simulink model "sampleModel1804_5_sub_sub"  (R2023a)
settings: Solver=VariableStepAuto  StartTime=0.0  StopTime=10.0  RelTol=1e-3
libraries: hdlsllib x5, simulink x1
settings Model: Creator=user1  LastModifiedBy=user1

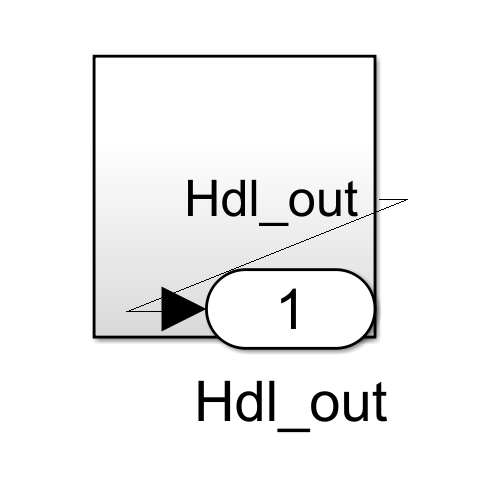
[thumbnail: Simulink's stored preview of the top-level diagram]
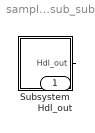
== system sampleModel1804_5_sub_sub ==
  Subsystem : Subsystem
  Hdl_out : Outport  OutDataTypeStr=uint8
  wires:
  Subsystem/1(Hdl_out) -> Hdl_out/1

== system sampleModel1804_5_sub_sub/Subsystem ==
  Subsystem : Subsystem
  Hdl_out : Outport  OutDataTypeStr=uint8

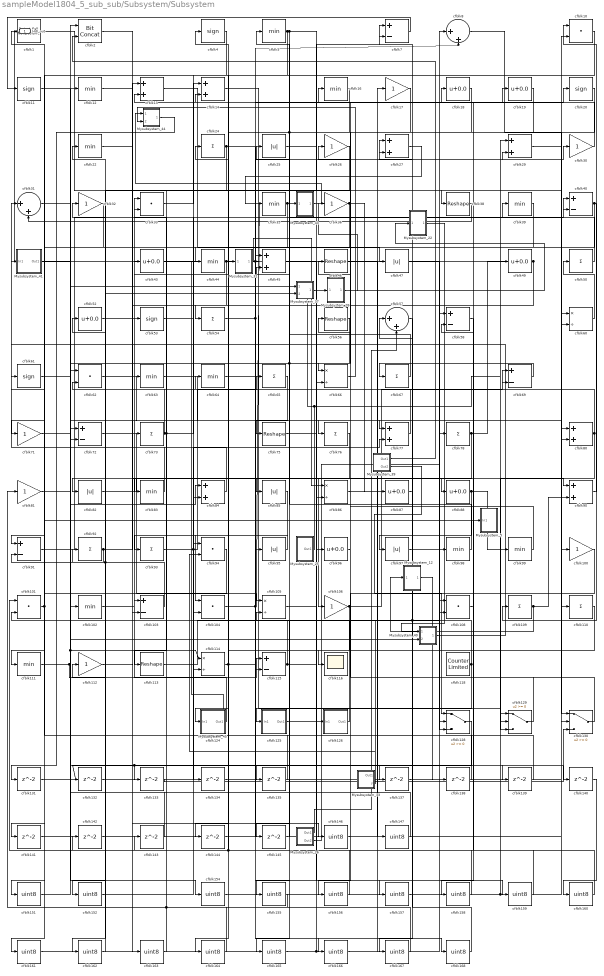
== system sampleModel1804_5_sub_sub/Subsystem/Subsystem ==
  Mysubsystem_12 : Subsystem  TreatAsAtomicUnit=on  RTWFcnName=Mysubsystem_12
      settings: RTWFcnNameOpts=User specified  RTWFileNameOpts=Use function name
  Mysubsystem_22 : Subsystem  TreatAsAtomicUnit=on  RTWFcnName=Mysubsystem_22
      settings: RTWFcnNameOpts=User specified  RTWFileNameOpts=Use function name
  Mysubsystem_25 : Subsystem  TreatAsAtomicUnit=on  RTWFcnName=Mysubsystem_25
      settings: RTWFcnNameOpts=User specified  RTWFileNameOpts=Use function name
  Mysubsystem_26 : Subsystem  TreatAsAtomicUnit=on  RTWFcnName=Mysubsystem_26
      settings: RTWFcnNameOpts=User specified  RTWFileNameOpts=Use function name
  Mysubsystem_28 : Subsystem  TreatAsAtomicUnit=on  RTWFcnName=Mysubsystem_28
      settings: RTWFcnNameOpts=User specified  RTWFileNameOpts=Use function name
  Mysubsystem_31 : Subsystem  TreatAsAtomicUnit=on  RTWFcnName=Mysubsystem_31
      settings: RTWFcnNameOpts=User specified  RTWFileNameOpts=Use function name
  Mysubsystem_33 : Subsystem  TreatAsAtomicUnit=on  RTWFcnName=Mysubsystem_33
      settings: RTWFcnNameOpts=User specified  RTWFileNameOpts=Use function name
  Mysubsystem_37 : Subsystem  TreatAsAtomicUnit=on  RTWFcnName=Mysubsystem_37
      settings: RTWFcnNameOpts=User specified  RTWFileNameOpts=Use function name
  Mysubsystem_39 : Subsystem  TreatAsAtomicUnit=on  RTWFcnName=Mysubsystem_39
      settings: RTWFcnNameOpts=User specified  RTWFileNameOpts=Use function name
  Mysubsystem_40 : Subsystem  TreatAsAtomicUnit=on  RTWFcnName=Mysubsystem_40
      settings: RTWFcnNameOpts=User specified  RTWFileNameOpts=Use function name
  Mysubsystem_41 : Subsystem  TreatAsAtomicUnit=on  RTWFcnName=Mysubsystem_41
      settings: RTWFcnNameOpts=User specified  RTWFileNameOpts=Use function name
  Mysubsystem_43 : Subsystem  TreatAsAtomicUnit=on  RTWFcnName=Mysubsystem_43
      settings: RTWFcnNameOpts=User specified  RTWFileNameOpts=Use function name
  Mysubsystem_44 : Subsystem  TreatAsAtomicUnit=on  RTWFcnName=Mysubsystem_44
      settings: RTWFcnNameOpts=User specified  RTWFileNameOpts=Use function name
  Mysubsystem_45 : Subsystem  TreatAsAtomicUnit=on  RTWFcnName=Mysubsystem_45
      settings: RTWFcnNameOpts=User specified  RTWFileNameOpts=Use function name
  Mysubsystem_5 : Subsystem  TreatAsAtomicUnit=on  RTWFcnName=Mysubsystem_5
      settings: RTWFcnNameOpts=User specified  RTWFileNameOpts=Use function name
  cfblk1 : hdlsllib/Logic and Bit Operations/Detect Fall Nonpositive  vinit=0  OutDataTypeStr=uint8
  cfblk{10,33,62,94,101,104,108} (7 alike) : DotProduct  OutDataTypeStr=uint8
  cfblk{17,26,30,32,36,71,81,100,106,112} (10 alike) : Gain  OutDataTypeStr=uint8
  cfblk{5,12,16,22,35,39,44,63..64,83,98..99,102,111} (14 alike) : MinMax  OutDataTypeStr=uint8
  cfblk{7,40,58,69,72,91,103,115} (8 alike) : Sum  Inputs=+-  OutDataTypeStr=uint8
  cfblk{60,66,86,105,114} (5 alike) : Product  Inputs=*/  OutDataTypeStr=uint8  RndMeth=Zero  SaturateOnIntegerOverflow=on
  cfblk{24,50,54,65,67,73,76,78,92..93,109..110} (12 alike) : Sum  Inputs=+  OutDataTypeStr=uint8
  cfblk{4,11,20,53,61} (5 alike) : Signum
  cfblk{38,46,56,75,113} (5 alike) : Reshape
  cfblk116 : Scope
  cfblk118 : hdlsllib/Sources/Counter Limited  uplimit=7  tsamp=-1
  cfblk124 : Subsystem
      settings: LibrarySourceBlock=|
      | hdlsllib/Ports &
      | Subsystems/Subsystem
  cfblk125 : Subsystem
      settings: LibrarySourceBlock=|
      | hdlsllib/Ports &
      | Subsystems/Subsystem
  cfblk126 : Subsystem
      settings: LibrarySourceBlock=|
      | hdlsllib/Ports &
      | Subsystems/Subsystem
  cfblk128 : Switch  OutDataTypeStr=uint8  SaturateOnIntegerOverflow=off  InputSameDT=off
  cfblk129 : Switch  OutDataTypeStr=uint8  SaturateOnIntegerOverflow=off  InputSameDT=off
  cfblk{13..14,27,29,45,77,80,84,90} (9 alike) : Sum  OutDataTypeStr=uint8
  cfblk130 : Switch  OutDataTypeStr=uint8  SaturateOnIntegerOverflow=off  InputSameDT=off
  cfblk{131..135,137..145} (14 alike) : Delay  SampleTime=1
  cfblk{146..147,151..152,154..168} (19 alike) : DataTypeConversion  OutDataTypeStr=uint8  SaturateOnIntegerOverflow=off  RndMeth=Floor
  cfblk{18..19,43,49,52,87..88,96} (8 alike) : Bias  Bias=0.0  SaturateOnIntegerOverflow=off
  cfblk2 : hdlsllib/Logic and Bit Operations/Bit Concat  numInputs=2
  cfblk{25,47,82,85,95,97} (6 alike) : Abs  OutDataTypeStr=uint8  SaturateOnIntegerOverflow=off
  cfblk31 : Sum  Inputs=|++  OutDataTypeStr=uint8
  cfblk57 : Sum  Inputs=|++  OutDataTypeStr=uint8
  cfblk8 : Sum  Inputs=|++  OutDataTypeStr=uint8
  Hdl_out : Outport  OutDataTypeStr=uint8
  wires:
  Mysubsystem_45/1(Out1) -> Mysubsystem_31/1(In1)
  Mysubsystem_44/1(Out1) -> cfblk131/1
  cfblk66/1 -> Mysubsystem_44/2(In2)
  Mysubsystem_43/1(Out1) -> Mysubsystem_44/1(In1)
  cfblk27/1 -> Mysubsystem_43/1(In1)
  Mysubsystem_41/1(Out1) -> Mysubsystem_40/2(In2)
  Mysubsystem_40/1(Out1) -> Mysubsystem_41/1(In1)
  Mysubsystem_22/1(Out1) -> Mysubsystem_40/1(In1)
  Mysubsystem_39/2(Out2) -> cfblk128/1
  Mysubsystem_39/1(Out1) -> cfblk2/2
  Mysubsystem_37/1(Out1) -> Mysubsystem_22/1(In1)
  cfblk31/1 -> Mysubsystem_37/1(In1)
  Mysubsystem_33/2(y) -> cfblk101/2
  Mysubsystem_33/1(Out1) -> cfblk94/2
  Mysubsystem_31/1(Out1) -> cfblk86/1
  Mysubsystem_28/1(Out1) -> cfblk36/1
  Mysubsystem_26/2(Out2) -> cfblk78/1
  Mysubsystem_26/1(Out1) -> cfblk57/2
  Mysubsystem_25/1(Out1) -> cfblk40/2, Mysubsystem_28/1(In1)
  Mysubsystem_12/1(Out1) -> cfblk138/1
  cfblk168/1 -> cfblk57/1
  cfblk64/1 -> cfblk168/1
  cfblk167/1 -> cfblk143/1, cfblk142/1
  cfblk166/1 -> cfblk17/1
  cfblk165/1 -> cfblk126/1(In1)
  cfblk17/1 -> cfblk165/1
  cfblk164/1 -> cfblk112/1
  cfblk163/1 -> cfblk33/2
  cfblk112/1 -> cfblk163/1
  cfblk162/1 -> cfblk32/1
  cfblk26/1 -> cfblk162/1
  cfblk161/1 -> cfblk108/2, cfblk96/1
  cfblk160/1 -> cfblk58/2
  cfblk140/1 -> cfblk160/1
  cfblk159/1 -> cfblk58/1
  cfblk158/1 -> cfblk62/2
  cfblk58/1 -> cfblk158/1
  cfblk157/1 -> cfblk100/1
  cfblk156/1 -> cfblk64/1, cfblk101/1
  cfblk155/1 -> cfblk81/1
  cfblk154/1 -> cfblk10/2, cfblk29/1
  cfblk152/1 -> cfblk94/1
  cfblk39/1 -> cfblk152/1
  cfblk151/1 -> cfblk102/1
  cfblk94/1 -> cfblk151/1
  cfblk147/1 -> cfblk2/1
  cfblk46/1 -> cfblk147/1
  cfblk146/1 -> cfblk108/1
  cfblk2/1 -> cfblk146/1
  cfblk145/1 -> cfblk105/2
  cfblk144/1 -> cfblk80/1
  cfblk110/1 -> cfblk144/1
  cfblk143/1 -> cfblk72/1
  cfblk142/1 -> cfblk45/1
  cfblk141/1 -> cfblk114/2
  cfblk139/1 -> cfblk1/1
  cfblk138/1 -> cfblk14/2
  cfblk137/1 -> cfblk129/1
  cfblk22/1 -> cfblk137/1
  cfblk135/1 -> cfblk62/1
  cfblk134/1 -> cfblk60/1
  cfblk43/1 -> cfblk134/1
  cfblk133/1 -> cfblk130/3
  cfblk132/1 -> cfblk115/2
  cfblk131/1 -> cfblk130/2
  cfblk63/1 -> cfblk95/1
  cfblk73/1 -> cfblk40/1, cfblk113/1, cfblk63/1
  cfblk45/1 -> cfblk129/2
  cfblk65/1 -> cfblk75/1
  cfblk100/1 -> cfblk156/1
  cfblk114/1 -> cfblk24/1, cfblk157/1
  cfblk101/1 -> Mysubsystem_5/1(In1), cfblk141/1
  cfblk97/1 -> cfblk98/1
  cfblk87/1 -> cfblk27/2
  cfblk24/1 -> cfblk83/1, cfblk140/1
  cfblk113/1 -> cfblk8/1
  cfblk95/1 -> cfblk93/1
  cfblk25/1 -> cfblk29/2
  cfblk50/1 -> cfblk25/1
  cfblk80/1 -> cfblk4/1, cfblk129/3
  cfblk98/1 -> cfblk45/2
  cfblk109/1 -> Mysubsystem_12/1(In1), cfblk90/2
  cfblk105/1 -> cfblk20/1
  cfblk38/1 -> cfblk31/2
  cfblk32/1 -> cfblk161/1
  cfblk57/1 -> cfblk167/1
  cfblk53/1 -> cfblk88/1
  cfblk11/1 -> cfblk77/1
  cfblk52/1 -> cfblk86/2
  cfblk128/1 -> cfblk132/1, cfblk133/1
  cfblk125/1(Out1) -> cfblk66/2
  cfblk29/1 -> cfblk130/1
  cfblk67/1 -> cfblk5/1
  cfblk71/1 -> cfblk12/1
  cfblk82/1 -> cfblk90/1
  cfblk77/1 -> cfblk22/1
  cfblk19/1 -> cfblk54/1
  cfblk8/1 -> cfblk110/1
  cfblk1/1 -> cfblk60/2
  cfblk88/1 -> cfblk97/1, cfblk99/1
  cfblk99/1 -> cfblk46/1
  cfblk12/1 -> cfblk53/1
  cfblk106/1 -> cfblk69/2, cfblk116/1
  cfblk84/1 -> cfblk73/1
  cfblk90/1 -> cfblk10/1
  cfblk124/1(Out1) -> cfblk103/1
  cfblk10/1 -> cfblk124/1(In1)
  cfblk60/1 -> cfblk50/1
  cfblk93/1 -> cfblk65/1, cfblk77/2
  cfblk96/1 -> cfblk56/1
  cfblk40/1 -> cfblk109/1, cfblk91/1
  cfblk86/1 -> cfblk69/1
  cfblk103/1 -> Mysubsystem_37/2(In2), cfblk61/1
  cfblk47/1 -> cfblk128/3
  cfblk115/1 -> cfblk92/1, cfblk159/1
  cfblk72/1 -> cfblk105/1
  cfblk33/1 -> cfblk14/1
  cfblk49/1 -> cfblk104/2, Hdl_out/1
  cfblk16/1 -> cfblk85/1
  cfblk111/1 -> cfblk115/1, cfblk84/1
  cfblk18/1 -> cfblk66/1
  cfblk76/1 -> cfblk106/1
  cfblk44/1 -> cfblk128/2, cfblk8/2, cfblk103/2
  cfblk78/1 -> cfblk82/1, cfblk49/1
  cfblk69/1 -> cfblk67/1
  cfblk30/1 -> cfblk13/2
  cfblk4/1 -> cfblk71/1
  cfblk56/1 -> cfblk72/2, cfblk135/1
  cfblk129/1 -> cfblk26/1
  cfblk85/1 -> cfblk104/1
  cfblk81/1 -> cfblk154/1
  cfblk5/1 -> cfblk38/1, cfblk125/1(In1), cfblk84/2
  cfblk7/1 -> cfblk11/1
  cfblk75/1 -> cfblk7/1
  cfblk36/1 -> cfblk44/1, cfblk87/1
  cfblk61/1 -> cfblk114/1, cfblk139/1
  cfblk108/1 -> cfblk18/1
  cfblk54/1 -> cfblk30/1, cfblk166/1
  cfblk83/1 -> cfblk31/1
  cfblk20/1 -> cfblk145/1, cfblk164/1
  cfblk62/1 -> cfblk80/2
  cfblk118/1 -> cfblk52/1, cfblk7/2, cfblk155/1
  cfblk35/1 -> cfblk27/1, cfblk111/1
  cfblk92/1 -> cfblk13/1, cfblk91/2
  cfblk91/1 -> cfblk39/1
  cfblk130/1 -> cfblk16/1
  cfblk104/1 -> cfblk35/1, cfblk19/1
  cfblk102/1 -> cfblk43/1
  cfblk126/1(Out1) -> cfblk33/1
  cfblk14/1 -> cfblk76/1
  cfblk13/1 -> cfblk47/1

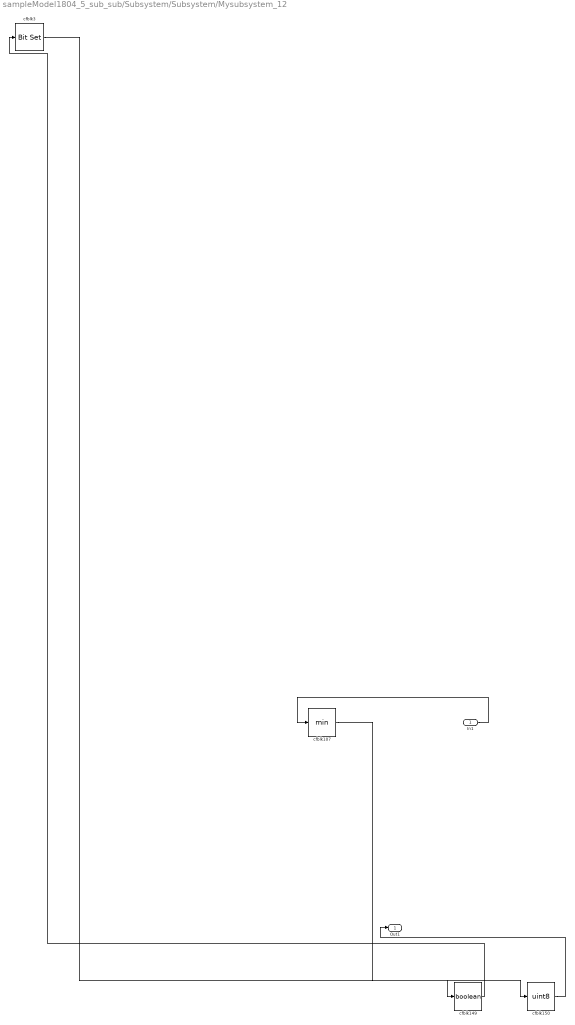
== system sampleModel1804_5_sub_sub/Subsystem/Subsystem/Mysubsystem_12 ==
  In1 : Inport
  cfblk107 : MinMax
  cfblk149 : DataTypeConversion  OutDataTypeStr=boolean  SaturateOnIntegerOverflow=off  RndMeth=Floor
  cfblk150 : DataTypeConversion  OutDataTypeStr=uint8  SaturateOnIntegerOverflow=off  RndMeth=Floor
  cfblk3 : simulink/Logic and Bit Operations/Bit Set  iBit=0
      settings: LibrarySourceBlock=|
      | hdlsllib/Logic and Bit
      | Operations/Bit Set
  Out1 : Outport
  wires:
  cfblk150/1 -> Out1/1
  cfblk3/1 -> cfblk150/1
  cfblk149/1 -> cfblk3/1
  cfblk107/1 -> cfblk149/1
  In1/1 -> cfblk107/1

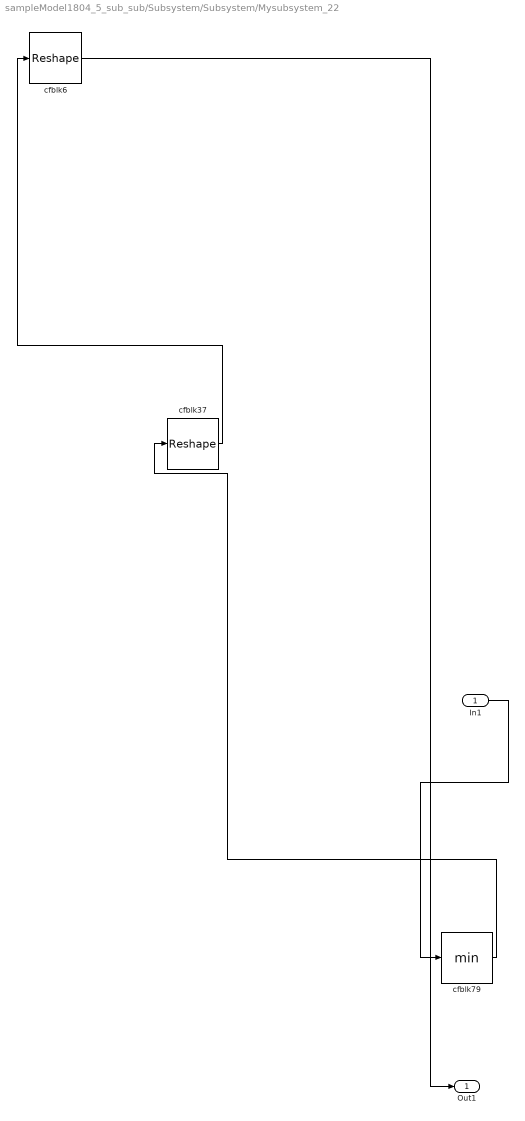
== system sampleModel1804_5_sub_sub/Subsystem/Subsystem/Mysubsystem_22 ==
  In1 : Inport
  cfblk37 : Reshape
  cfblk6 : Reshape
  cfblk79 : MinMax
  Out1 : Outport
  wires:
  cfblk37/1 -> cfblk6/1
  cfblk79/1 -> cfblk37/1
  In1/1 -> cfblk79/1
  cfblk6/1 -> Out1/1

== system sampleModel1804_5_sub_sub/Subsystem/Subsystem/Mysubsystem_25 ==
  cfblk123 : Constant  SampleTime=-1
  cfblk68 : Reshape
  Out1 : Outport
  wires:
  cfblk123/1 -> cfblk68/1
  cfblk68/1 -> Out1/1

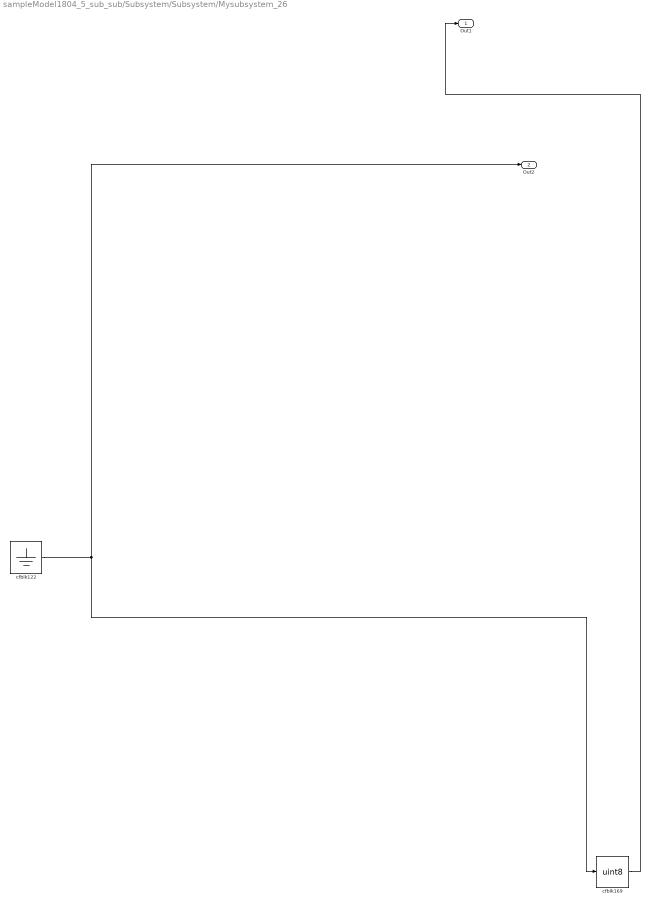
== system sampleModel1804_5_sub_sub/Subsystem/Subsystem/Mysubsystem_26 ==
  cfblk122 : Ground
  cfblk169 : DataTypeConversion  OutDataTypeStr=uint8  SaturateOnIntegerOverflow=off  RndMeth=Floor
  Out1 : Outport
  Out2 : Outport  Port=2
  wires:
  cfblk122/1 -> Out2/1, cfblk169/1
  cfblk169/1 -> Out1/1

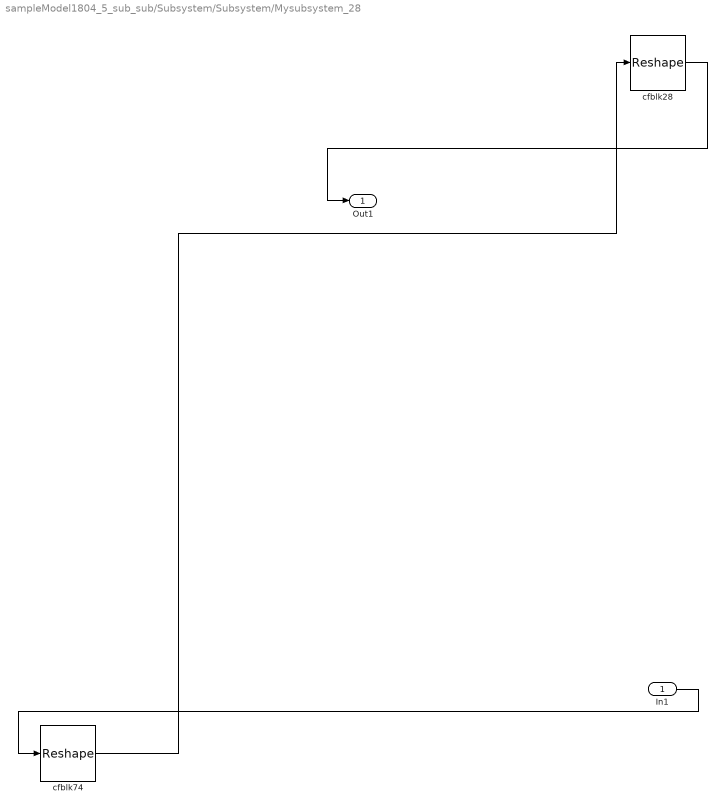
== system sampleModel1804_5_sub_sub/Subsystem/Subsystem/Mysubsystem_28 ==
  In1 : Inport
  cfblk28 : Reshape
  cfblk74 : Reshape
  Out1 : Outport
  wires:
  cfblk74/1 -> cfblk28/1
  cfblk28/1 -> Out1/1
  In1/1 -> cfblk74/1

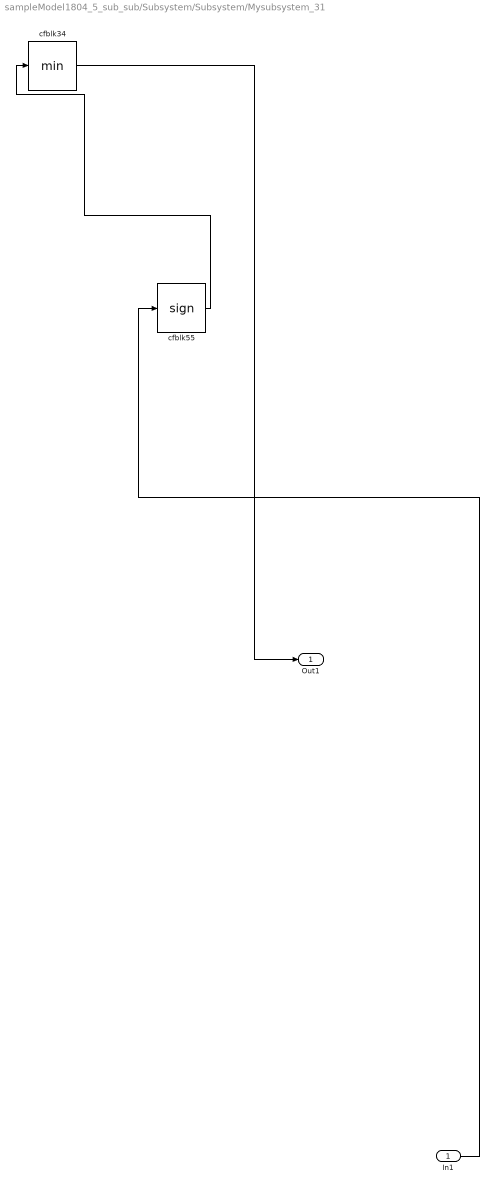
== system sampleModel1804_5_sub_sub/Subsystem/Subsystem/Mysubsystem_31 ==
  In1 : Inport
  cfblk34 : MinMax
  cfblk55 : Signum
  Out1 : Outport
  wires:
  In1/1 -> cfblk55/1
  cfblk55/1 -> cfblk34/1
  cfblk34/1 -> Out1/1

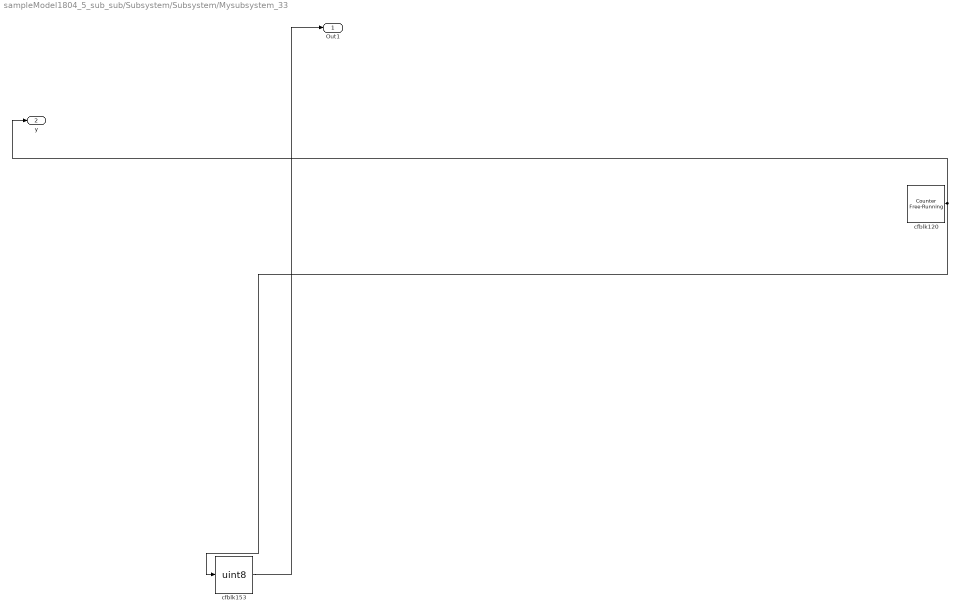
== system sampleModel1804_5_sub_sub/Subsystem/Subsystem/Mysubsystem_33 ==
  cfblk120 : hdlsllib/Sources/Counter Free-Running  NumBits=16  tsamp=-1
  cfblk153 : DataTypeConversion  OutDataTypeStr=uint8  SaturateOnIntegerOverflow=off  RndMeth=Floor
  Out1 : Outport
  y : Outport  Port=2
  wires:
  cfblk120/1 -> y/1, cfblk153/1
  cfblk153/1 -> Out1/1

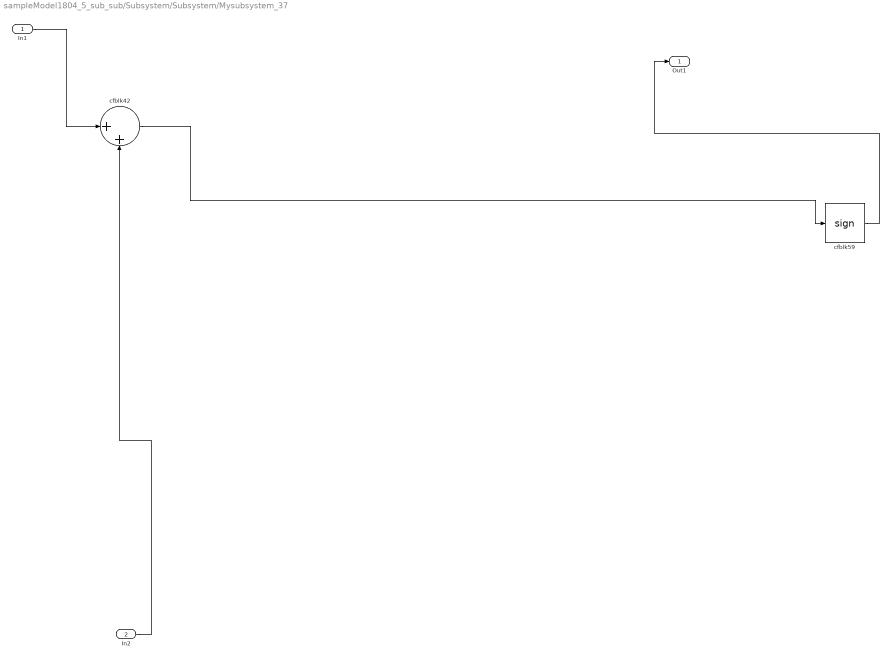
== system sampleModel1804_5_sub_sub/Subsystem/Subsystem/Mysubsystem_37 ==
  In1 : Inport
  In2 : Inport  Port=2
  cfblk42 : Sum  Inputs=|++
  cfblk59 : Signum
  Out1 : Outport
  wires:
  cfblk42/1 -> cfblk59/1
  In1/1 -> cfblk42/1
  cfblk59/1 -> Out1/1
  In2/1 -> cfblk42/2

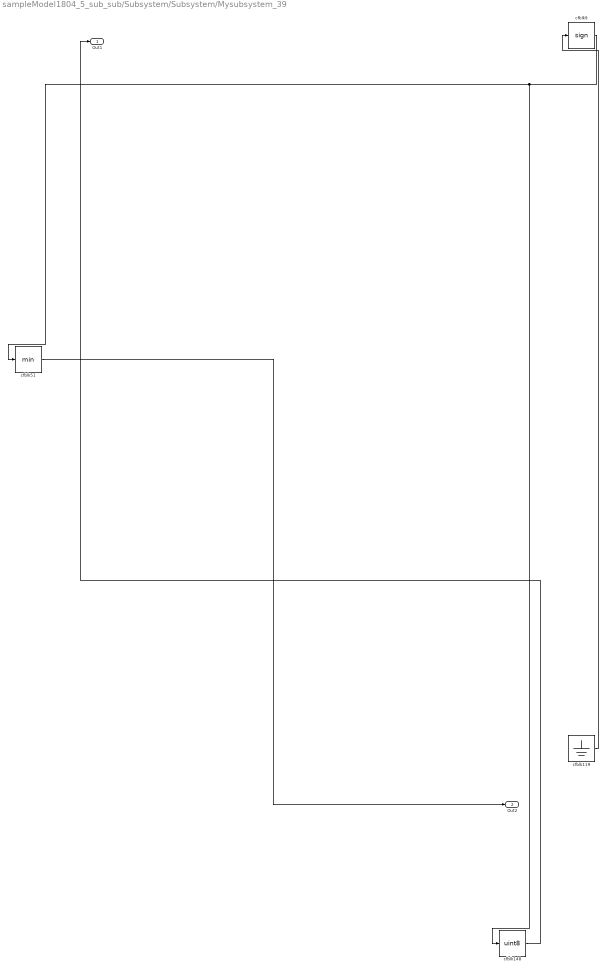
== system sampleModel1804_5_sub_sub/Subsystem/Subsystem/Mysubsystem_39 ==
  cfblk119 : Ground
  cfblk148 : DataTypeConversion  OutDataTypeStr=uint8  SaturateOnIntegerOverflow=off  RndMeth=Floor
  cfblk51 : MinMax
  cfblk9 : Signum
  Out1 : Outport
  Out2 : Outport  Port=2
  wires:
  cfblk119/1 -> cfblk9/1
  cfblk9/1 -> cfblk51/1, cfblk148/1
  cfblk51/1 -> Out2/1
  cfblk148/1 -> Out1/1

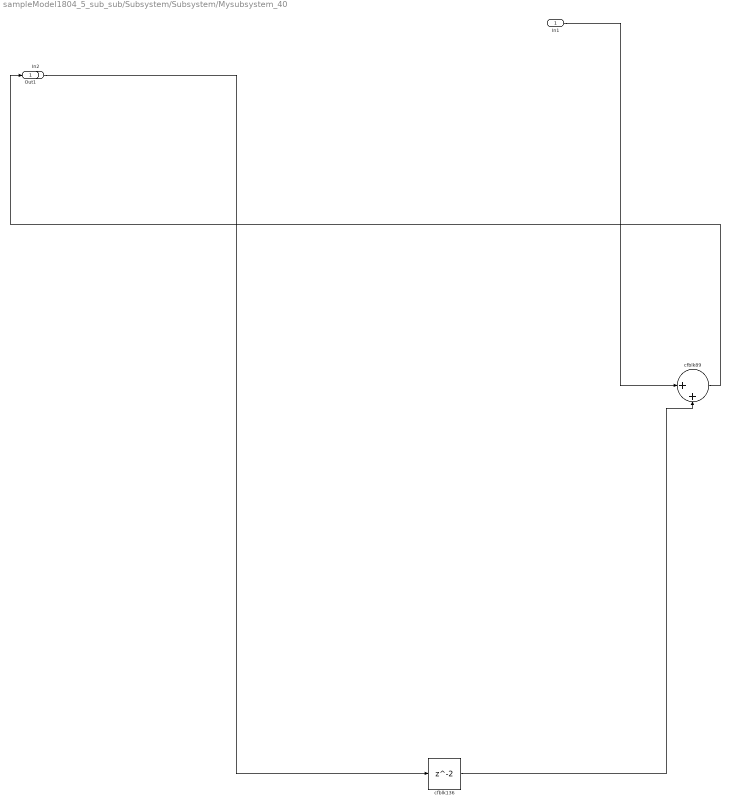
== system sampleModel1804_5_sub_sub/Subsystem/Subsystem/Mysubsystem_40 ==
  In1 : Inport
  In2 : Inport  Port=2
  cfblk136 : Delay  SampleTime=1
  cfblk89 : Sum  Inputs=|++
  Out1 : Outport
  wires:
  cfblk136/1 -> cfblk89/2
  In1/1 -> cfblk89/1
  In2/1 -> cfblk136/1
  cfblk89/1 -> Out1/1

== system sampleModel1804_5_sub_sub/Subsystem/Subsystem/Mysubsystem_41 ==
  In1 : Inport
  cfblk41 : MinMax
  Out1 : Outport
  wires:
  In1/1 -> cfblk41/1
  cfblk41/1 -> Out1/1

== system sampleModel1804_5_sub_sub/Subsystem/Subsystem/Mysubsystem_43 ==
  In1 : Inport
  cfblk23 : Abs  SaturateOnIntegerOverflow=off
  cfblk48 : Sum  Inputs=+
  Out1 : Outport
  wires:
  cfblk23/1 -> cfblk48/1
  cfblk48/1 -> Out1/1
  In1/1 -> cfblk23/1

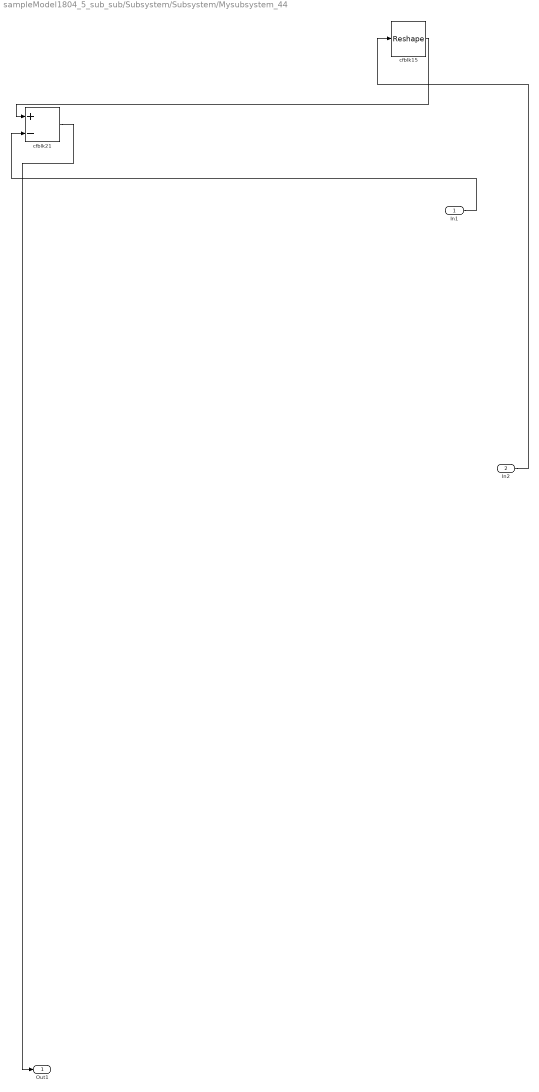
== system sampleModel1804_5_sub_sub/Subsystem/Subsystem/Mysubsystem_44 ==
  In1 : Inport
  In2 : Inport  Port=2
  cfblk15 : Reshape
  cfblk21 : Sum  Inputs=+-
  Out1 : Outport
  wires:
  cfblk21/1 -> Out1/1
  cfblk15/1 -> cfblk21/1
  In1/1 -> cfblk21/2
  In2/1 -> cfblk15/1

== system sampleModel1804_5_sub_sub/Subsystem/Subsystem/Mysubsystem_45 ==
  cfblk121 : hdlsllib/Sources/Counter Limited  uplimit=7  tsamp=-1
  cfblk127 : Subsystem
      settings: LibrarySourceBlock=|
      | hdlsllib/Ports &
      | Subsystems/Subsystem
  Out1 : Outport
  wires:
  cfblk121/1 -> cfblk127/1(In1)
  cfblk127/1(Out1) -> Out1/1

== system sampleModel1804_5_sub_sub/Subsystem/Subsystem/Mysubsystem_5 ==
  In1 : Inport
  cfblk117 : ToWorkspace  VariableName=simout  SaveFormat=Timeseries  SampleTime=-1
  cfblk70 : Signum
  wires:
  cfblk70/1 -> cfblk117/1
  In1/1 -> cfblk70/1

== system sampleModel1804_5_sub_sub/Subsystem/Subsystem/cfblk124 ==
  In1 : Inport
  Out1 : Outport
  wires:
  In1/1 -> Out1/1

== system sampleModel1804_5_sub_sub/Subsystem/Subsystem/cfblk125 ==
  In1 : Inport
  Out1 : Outport
  wires:
  In1/1 -> Out1/1

== system sampleModel1804_5_sub_sub/Subsystem/Subsystem/cfblk126 ==
  In1 : Inport
  Out1 : Outport
  wires:
  In1/1 -> Out1/1

== system sampleModel1804_5_sub_sub/Subsystem/Subsystem/Mysubsystem_45/cfblk127 ==
  In1 : Inport
  Out1 : Outport
  wires:
  In1/1 -> Out1/1
